simulink model "manning_test_nonlinear_difflink"  (R2022b)
settings: Solver=VariableStepAuto  StartTime=0.0  StopTime=5*34416  RelTol=1e-3
undefined symbols (not defined in the file): yd_ds
settings Model: Creator=chuan  LastModifiedBy=chuan

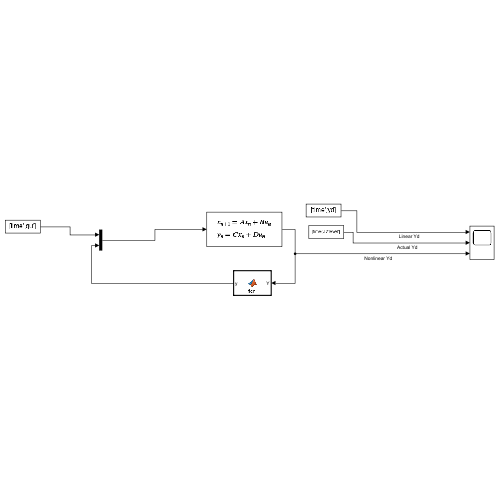
[thumbnail: Simulink's stored preview of the top-level diagram]
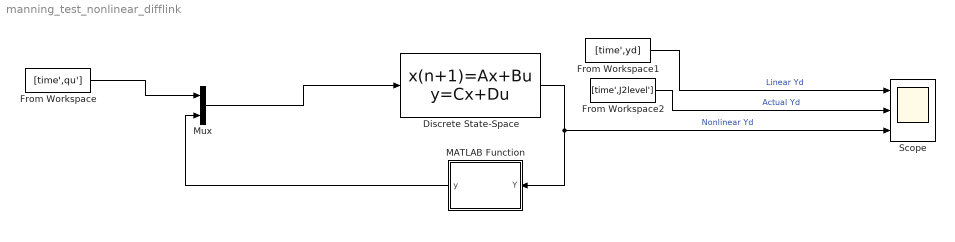
== system manning_test_nonlinear_difflink ==
  Discrete State-Space : DiscreteStateSpace  A=yd_ds.A  B=yd_ds.B  C=yd_ds.C  D=yd_ds.D  SampleTime=yd_ds.Ts
  From Workspace : FromWorkspace  VariableName=[time',qu']
  From Workspace1 : FromWorkspace  VariableName=[time',yd]
  From Workspace2 : FromWorkspace  VariableName=[time',J2level']
  MATLAB Function : MATLAB Function  TreatAsAtomicUnit=on
  Mux : Mux  Inputs=2
  Scope : Scope  NumInputPorts=3
  wires:
  Discrete State-Space/1 -> Scope/3, MATLAB Function/1(Y)  "Nonlinear Yd"
  MATLAB Function/1(y) -> Mux/2
  Mux/1 -> Discrete State-Space/1
  From Workspace/1 -> Mux/1
  From Workspace1/1 -> Scope/1  "Linear Yd"
  From Workspace2/1 -> Scope/2  "Actual Yd"

== matlab function manning_test_nonlinear_difflink/MATLAB Function ==
  data: Y input; y output
function y = fcn(Y)
n = 0.04;
Sb = 0.0025;
B=2;
% Sb = 0.0008;
% B = 8;
m = 1.5;

Y = max(Y,0);

y = (1/n)*(B*Y + m*Y.^2)*((B*Y + m*Y.^2)/(B + 2.*Y.*sqrt(1+m^2))).^(2/3) .* sqrt(Sb);
